simulink model "FCHEV_noDCbus"  (R2023a)
settings: Solver=ode23tb  StartTime=0.0  StopTime=20e3  MaxStep=1e-1  RelTol=1e-4
libraries: component_lib x10, slpidlib x1
settings Model: Creator=maxjo65  LastModifiedBy=maxjo65
settings OptimizationCC: ReuseModelBlockBuffer=off
settings DebuggingCC: UnconnectedInputMsg=warning  UnconnectedOutputMsg=warning  UnconnectedLineMsg=warning
settings ModelReferenceCC: EnableRefExpFcnMdlSchedulingChecks=on
settings RTWCC: DLArmComputeVersion=19.05

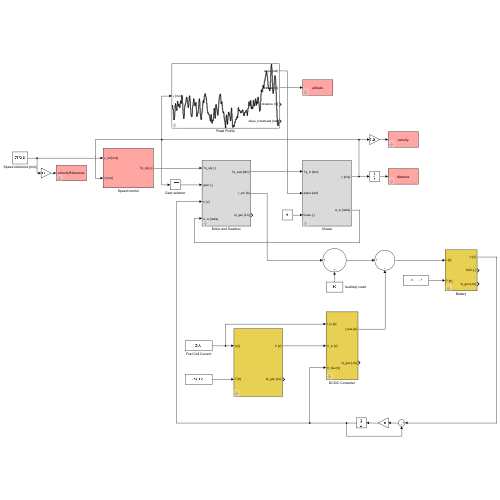
[thumbnail: Simulink's stored preview of the top-level diagram]
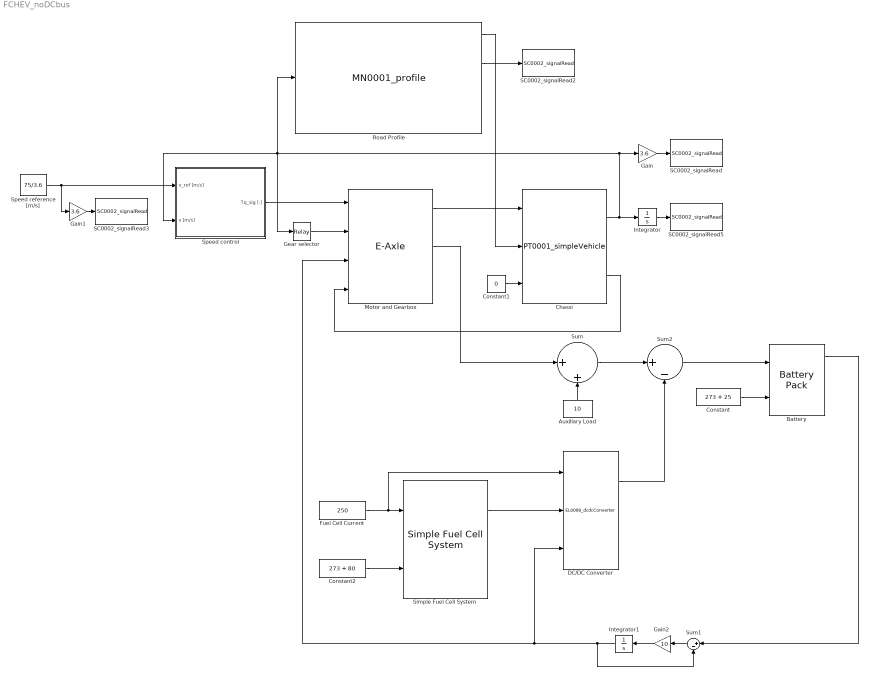
== system FCHEV_noDCbus ==
  Auxillary Load : Constant  Value=10
  Battery : component_lib/Battery Pack  SOC_0=0.5  Nx=120  Ny=180
  Chassi : component_lib/Powertrain/PT0001_simpleVehicle  m=40e3  r_w=0.5  A_f=10  C_d=0.5  rho_air=1.225  c_r0=0.0060  c_r1=2.3e-7  gain=600  v0=75/3.6  x0=0
  Constant : Constant  Value=273 + 25
  Constant1 : Constant  Value=0
  Constant2 : Constant  Value=273 + 80
  DC/DC Converter : component_lib/Electrochemistry/EL0008_dcdcConverter  eta_up=0.99  eta_down=0.99
  Fuel Cell Current : Constant  Value=250
  Gain : Gain  Gain=3.6
  Gain1 : Gain  Gain=3.6
  Gain2 : Gain  Gain=10
  Gear selector : Relay  OnSwitchValue=22  OffSwitchValue=21.5  OnOutputValue=4  OffOutputValue=3
  Integrator : Integrator
  Integrator1 : Integrator  InitialCondition=700
  Motor and Gearbox : component_lib/E-Axle  n=3  V_nom=700
  Road Profile : component_lib/Mission/MN0001_profile  profile=Sodertalje_Norrkoping.mat  x0=0  N_lookahead=100
  SC0002_signalRead : component_lib/Data & Control/SC0002_signalRead  SigName=velocity
  SC0002_signalRead2 : component_lib/Data & Control/SC0002_signalRead  SigName=altitude
  SC0002_signalRead3 : component_lib/Data & Control/SC0002_signalRead  SigName=velocityReference
  SC0002_signalRead5 : component_lib/Data & Control/SC0002_signalRead  SigName=distance
  Simple Fuel Cell System : component_lib/Simple Fuel Cell System  n_st=2  n=375
  Speed control : Subsystem
  Speed reference [m/s] : Constant  Value=75/3.6
  Sum : Sum  Inputs=|++
  Sum1 : Sum  Inputs=|+-
  Sum2 : Sum  Inputs=|+-
  wires:
  Motor and Gearbox/1 -> Chassi/1
  Chassi/2 -> Motor and Gearbox/4
  Road Profile/1 -> Chassi/2
  Chassi/1 -> Integrator/1, Gain/1, Speed control/2(v [m/s]), Road Profile/1, Gear selector/1
  Speed reference [m/s]/1 -> Gain1/1, Speed control/1(v_ref [m/s])
  Speed control/1(Tq_sig [-]) -> Motor and Gearbox/1
  Gear selector/1 -> Motor and Gearbox/2
  Integrator/1 -> SC0002_signalRead5/1
  Gain/1 -> SC0002_signalRead/1
  Road Profile/2 -> SC0002_signalRead2/1
  Gain1/1 -> SC0002_signalRead3/1
  Constant1/1 -> Chassi/3
  Constant2/1 -> Simple Fuel Cell System/2
  Constant/1 -> Battery/2
  Auxillary Load/1 -> Sum/2
  Fuel Cell Current/1 -> Simple Fuel Cell System/1, DC/DC Converter/1
  Integrator1/1 -> DC/DC Converter/3, Motor and Gearbox/3, Sum1/2
  Sum/1 -> Sum2/1
  Simple Fuel Cell System/1 -> DC/DC Converter/2
  DC/DC Converter/1 -> Sum2/2
  Sum2/1 -> Battery/1
  Battery/1 -> Sum1/1
  Sum1/1 -> Gain2/1
  Gain2/1 -> Integrator1/1
  Motor and Gearbox/2 -> Sum/1

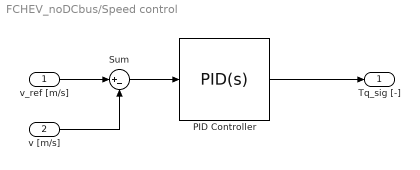
== system FCHEV_noDCbus/Speed control ==
  v_ref [m/s] : Inport
  v [m/s] : Inport  Port=2
  PID Controller : slpidlib/PID Controller  Controller=PID  Form=Parallel  TimeDomain=Continuous-time  UseExternalTs=off  SampleTime=-1  IntegratorMethod=Forward Euler  FilterMethod=Forward Euler  ControllerParametersSource=internal  P=10  I=1e-1  UseKiTs=off  D=0  N=100  UseFilter=on  TunerSelectOption=Transfer Function Based (PID Tuner App)  ZeroCross=off  InitialConditionSource=internal  InitialConditionForIntegrator=0  InitialConditionForFilter=0  DifferentiatorICPrevScaledInput=0  ExternalReset=none  TrackingMode=off  Kt=1  LimitOutput=on  SatLimitsSource=internal  UpperSaturationLimit=1  LowerSaturationLimit=-1  LinearizeAsGain=on  AntiWindupMode=clamping  Kb=1  LimitIntegrator=off  UpperIntegratorSaturationLimit=inf  LowerIntegratorSaturationLimit=-inf  POutMin=[]  POutMax=[]  IOutMin=[]  IOutMax=[]  DOutMin=[]  DOutMax=[]  NOutMin=[]  NOutMax=[]  SumOutMin=[]  SumOutMax=[]  SaturationOutMin=[]  SaturationOutMax=[]  PParamMin=[]  PParamMax=[]  IParamMin=[]  IParamMax=[]  DParamMin=[]  DParamMax=[]  NParamMin=[]  NParamMax=[]  KbParamMin=[]  KbParamMax=[]  KtParamMin=[]  KtParamMax=[]  KbOutMin=[]  KbOutMax=[]  KtOutMin=[]  KtOutMax=[]  IntegratorOutMin=[]  IntegratorOutMax=[]  FilterOutMin=[]  FilterOutMax=[]  SumI1OutMin=[]  SumI1OutMax=[]  SumI2OutMin=[]  SumI2OutMax=[]  SumI3OutMin=[]  SumI3OutMax=[]  SumI4OutMin=[]  SumI4OutMax=[]  SumDOutMin=[]  SumDOutMax=[]  DifferentiatorOutMin=[]  DifferentiatorOutMax=[]  FilterDiffOutCoefMin=[]  FilterDiffOutCoefMax=[]  ReciprocalOutMin=[]  ReciprocalOutMax=[]  SumDenOutMin=[]  SumDenOutMax=[]  SumNumOutMin=[]  SumNumOutMax=[]  DivideOutMin=[]  DivideOutMax=[]  UdiffTsProdOutMin=[]  UdiffTsProdOutMax=[]  NTsProdOutMin=[]  NTsProdOutMax=[]  UintegralTsProdOutMin=[]  UintegralTsProdOutMax=[]  UngainTsProdOutMin=[]  UngainTsProdOutMax=[]  ClampingZeroOutDataTypeStr=Inherit: Inherit via back propagation  ClampingZeroOutMin=[]  ClampingZeroOutMax=[]  FilterDenConstantOutDataTypeStr=Inherit: Inherit via back propagation  FilterDenConstantOutMin=[]  FilterDenConstantOutMax=[]  PCopyOutDataTypeStr=Inherit: Inherit via back propagation  PCopyOutMin=[]  PCopyOutMax=[]  NCopyOutDataTypeStr=Inherit: Inherit via back propagation  NCopyOutMin=[]  NCopyOutMax=[]  IntegratorContinuousStateAttributes=''  IntegratorStateMustResolveToSignalObject=off  IntegratorRTWStateStorageClass=Auto  FilterContinuousStateAttributes=''  FilterStateMustResolveToSignalObject=off  FilterRTWStateStorageClass=Auto  ParallelPVariant=InternalParameters  IdealPVariant=Disabled  IVariant=InternalParameters  DVariant=InternalParameters  IntegratorVariant=Continuous  SatVariant=Enabled  AWVariant=ContClampingParallel  PCopyVariant=Disabled  TRVariant=Disabled  FdbkBlocksVariant=Forward  IdealPFdbkVariant=Disabled  SatFdbkVariant=Disabled  DerivativeFilterVariant=ContFilter  NVariant=InternalParameters  NCopyVariant=Disabled  FilterICVariant=InternalICsFilter  IntegratorICVariant=InternalICs  ExternalResetVariant=Disabled  TRSumVariant=Passthrough  SumFdbkVariant=Disabled  SumVariant=Sum_PID  TsampFilterVariant=InternalTs  TsampNgainVariant=Passthrough  TsampIntegralVariant=Disabled_SignalSpec  ExternalSaturationOutDataTypeStr=Inherit: Same as second input
  Sum : Sum  Inputs=|+-
  Tq_sig [-] : Outport
  wires:
  PID Controller/1 -> Tq_sig [-]/1
  Sum/1 -> PID Controller/1
  v_ref [m/s]/1 -> Sum/1
  v [m/s]/1 -> Sum/2
